simulink model "motor_control_model_mk4"  (R2023b)
settings: Solver=FixedStepAuto  StartTime=0.0  StopTime=80  FixedStep=0.0001  RelTol=1e-5
values from neighbouring files (symbols this model uses):
  A = 1    [paramterters.mat]    (also in set_parameters.m)
  batt_volt = 144    [paramterters.mat]    (also in set_parameters.m)
  C_d = 0.7    [paramterters.mat]    (also in set_parameters.m)
  fric_coeff = 0.03    [paramterters.mat]    (also in set_parameters.m)
  g = 9.81    [paramterters.mat]    (also in set_parameters.m)
  gear_ratio = 4.2    [paramterters.mat]    (also in set_parameters.m)
  grad_degrees = 0    [paramterters.mat]    (also in set_parameters.m)
  J_net = 1.34126984127    [paramterters.mat]    (also in set_parameters.m)
  K_t = 0.3472    [paramterters.mat]    (also in set_parameters.m)
  mass_vehicle = 350    [paramterters.mat]    (also in set_parameters.m)
  motor_eff = 0.85    [paramterters.mat]    (also in set_parameters.m)
  pc_eff = 0.9    [paramterters.mat]    (also in set_parameters.m)
  R_a = 0.02    [paramterters.mat]    (also in set_parameters.m)
  rho = 1.29    [paramterters.mat]    (also in set_parameters.m)
  wheel_radius = 0.26    [paramterters.mat]    (also in set_parameters.m)
libraries: slpidlib x3, spsPWMGeneratorDCDCLib x1
settings Model: Creator=shank  LastModifiedBy=shank

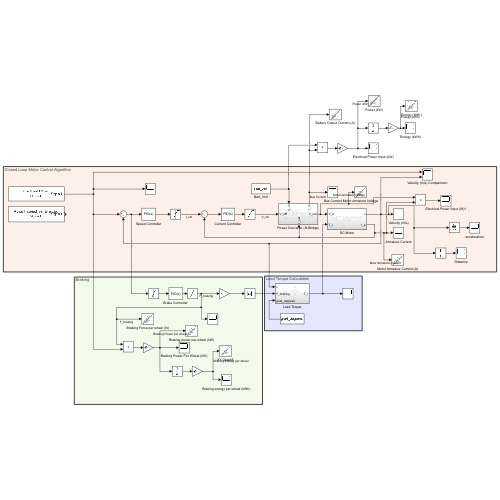
[thumbnail: Simulink's stored preview of the top-level diagram]
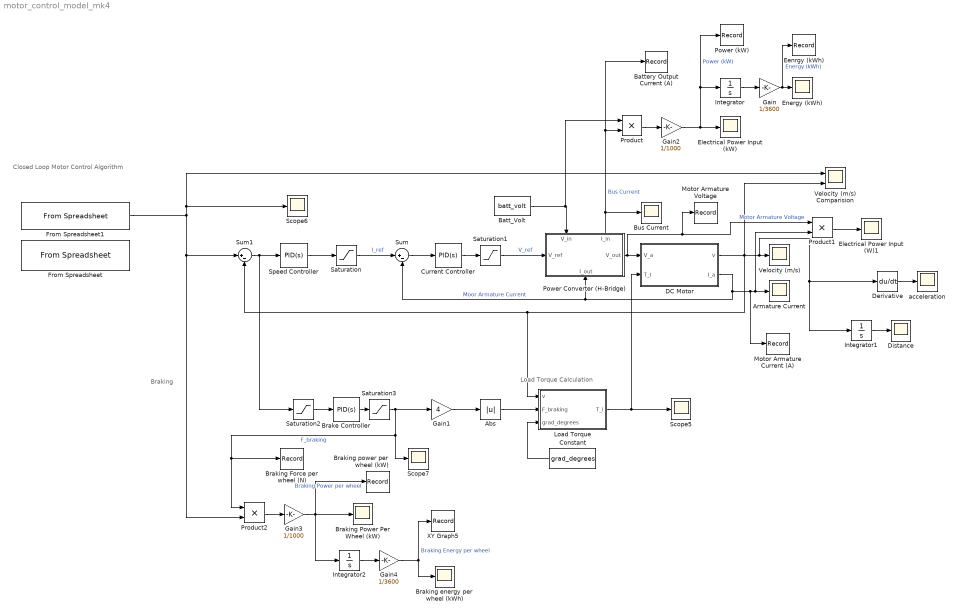
== system motor_control_model_mk4 ==
  note: Closed Loop Motor Control Algorithm
  note: Load Torque Calculation
  note: Braking
  Abs : Abs  SaturateOnIntegerOverflow=off
  Armature Current : Scope
  Batt_Volt : Constant  Value=batt_volt
  Battery Output Current (A) : Record  FileSettingsInternal="{\"entries\":[{\"content\":{\"excelSettings\":{\"content\":{},\"type\":\"Streamout.ExcelSettings\"}},\"type\":\"Streamout.FileSettingStorage\",\"uuid\":\"\"}],\"packageUris\":[\"http:\\/\\/schema.mathworks.com\\/mf0\\/streamout_blocks\\/R2020a\"],\"version\":\"1.0\"}"  Layout=[1 1]  SignalsInternal="{\"entries\":[{\"content\":{\"signals\":[{\"content\":{\"blockPath\":[],\"dimensions\":[1],\"domain\":\"\",\"lineColor\":\"#77ac30\",\"plots\":[1],\"port\":1,\"sid\":[\"\"],\"signalID\":369,\"signalName\":\"Bus Current\"},\"type\":\"RecordBlkView.Signal\",\"uuid\":\"\"}]},\"type\":\"RecordBlkView.InputSignals\",\"uuid\":\"\"}],\"packageUris\":[\"http:\\/\\/schema.mathworks.com\\/mf0\\/streamout_blocks\\/R2020a\"],\"version\":\"1.0\"}"  CompatibilityTag=XY
  Brake Controller : slpidlib/PID Controller  Controller=PID  Form=Parallel  TimeDomain=Continuous-time  UseExternalTs=off  SampleTime=-1  IntegratorMethod=Forward Euler  FilterMethod=Forward Euler  ControllerParametersSource=internal  P=500  I=0  UseKiTs=off  D=10  N=100  UseFilter=on  TunerSelectOption=Transfer Function Based (PID Tuner App)  InitialConditionSource=internal  InitialConditionForIntegrator=0  InitialConditionForFilter=0  DifferentiatorICPrevScaledInput=0  ExternalReset=none  TrackingMode=off  Kt=1  LimitOutput=off  SatLimitsSource=internal  UpperSaturationLimit=inf  LowerSaturationLimit=-inf  LinearizeAsGain=on  AntiWindupMode=none  Kb=1  LimitIntegrator=off  UpperIntegratorSaturationLimit=inf  LowerIntegratorSaturationLimit=-inf  POutMin=[]  POutMax=[]  IOutMin=[]  IOutMax=[]  DOutMin=[]  DOutMax=[]  NOutMin=[]  NOutMax=[]  SumOutMin=[]  SumOutMax=[]  SaturationOutMin=[]  SaturationOutMax=[]  PParamMin=[]  PParamMax=[]  IParamMin=[]  IParamMax=[]  DParamMin=[]  DParamMax=[]  NParamMin=[]  NParamMax=[]  KbParamMin=[]  KbParamMax=[]  KtParamMin=[]  KtParamMax=[]  KbOutMin=[]  KbOutMax=[]  KtOutMin=[]  KtOutMax=[]  IntegratorOutMin=[]  IntegratorOutMax=[]  FilterOutMin=[]  FilterOutMax=[]  SumI1OutMin=[]  SumI1OutMax=[]  SumI2OutMin=[]  SumI2OutMax=[]  SumI3OutMin=[]  SumI3OutMax=[]  SumI4OutMin=[]  SumI4OutMax=[]  SumDOutMin=[]  SumDOutMax=[]  DifferentiatorOutMin=[]  DifferentiatorOutMax=[]  FilterDiffOutCoefMin=[]  FilterDiffOutCoefMax=[]  ReciprocalOutMin=[]  ReciprocalOutMax=[]  SumDenOutMin=[]  SumDenOutMax=[]  SumNumOutMin=[]  SumNumOutMax=[]  DivideOutMin=[]  DivideOutMax=[]  UdiffTsProdOutMin=[]  UdiffTsProdOutMax=[]  NTsProdOutMin=[]  NTsProdOutMax=[]  UintegralTsProdOutMin=[]  UintegralTsProdOutMax=[]  UngainTsProdOutMin=[]  UngainTsProdOutMax=[]  ClampingZeroOutDataTypeStr=Inherit: Inherit via back propagation  ClampingZeroOutMin=[]  ClampingZeroOutMax=[]  FilterDenConstantOutDataTypeStr=Inherit: Inherit via back propagation  FilterDenConstantOutMin=[]  FilterDenConstantOutMax=[]  PCopyOutDataTypeStr=Inherit: Inherit via back propagation  PCopyOutMin=[]  PCopyOutMax=[]  NCopyOutDataTypeStr=Inherit: Inherit via back propagation  NCopyOutMin=[]  NCopyOutMax=[]  IntegratorContinuousStateAttributes=''  IntegratorStateMustResolveToSignalObject=off  IntegratorRTWStateStorageClass=Auto  FilterContinuousStateAttributes=''  FilterStateMustResolveToSignalObject=off  FilterRTWStateStorageClass=Auto  ParallelPVariant=InternalParameters  IdealPVariant=Disabled  IVariant=InternalParameters  DVariant=InternalParameters  IntegratorVariant=Continuous  SatVariant=Disabled  AWVariant=Passthrough  PCopyVariant=Disabled  TRVariant=Disabled  FdbkBlocksVariant=Forward  IdealPFdbkVariant=Disabled  SatFdbkVariant=Disabled  DerivativeFilterVariant=ContFilter  NVariant=InternalParameters  NCopyVariant=Disabled  FilterICVariant=InternalICsFilter  IntegratorICVariant=InternalICs  ExternalResetVariant=Disabled  TRSumVariant=Passthrough  SumFdbkVariant=Disabled  SumVariant=Sum_PID  TsampFilterVariant=InternalTs  TsampNgainVariant=Passthrough  TsampIntegralVariant=Disabled_SignalSpec  ExternalSaturationOutDataTypeStr=Inherit: Same as second input
  Braking Force per wheel (N) : Record  FileSettingsInternal="{\"entries\":[{\"content\":{\"excelSettings\":{\"content\":{},\"type\":\"Streamout.ExcelSettings\"}},\"type\":\"Streamout.FileSettingStorage\",\"uuid\":\"\"}],\"packageUris\":[\"http:\\/\\/schema.mathworks.com\\/mf0\\/streamout_blocks\\/R2020a\"],\"version\":\"1.0\"}"  Layout=[1 1]  SignalsInternal="{\"entries\":[{\"content\":{\"signals\":[{\"content\":{\"blockPath\":[],\"dimensions\":[1],\"domain\":\"\",\"lineColor\":\"#4dbeee\",\"plots\":[1],\"port\":1,\"sid\":[\"\"],\"signalID\":373,\"signalName\":\"F_braking\"},\"type\":\"RecordBlkView.Signal\",\"uuid\":\"\"}]},\"type\":\"RecordBlkView.InputSignals\",\"uuid\":\"\"}],\"packageUris\":[\"http:\\/\\/schema.mathworks.com\\/mf0\\/streamout_blocks\\/R2020a\"],\"version\":\"1.0\"}"  CompatibilityTag=XY
  Braking Power Per Wheel (kW) : Scope
  Braking energy per wheel (kWh) : Scope
  Braking power per wheel (kW) : Record  FileSettingsInternal="{\"entries\":[{\"content\":{\"excelSettings\":{\"content\":{},\"type\":\"Streamout.ExcelSettings\"}},\"type\":\"Streamout.FileSettingStorage\",\"uuid\":\"\"}],\"packageUris\":[\"http:\\/\\/schema.mathworks.com\\/mf0\\/streamout_blocks\\/R2020a\"],\"version\":\"1.0\"}"  Layout=[1 1]  SignalsInternal="{\"entries\":[{\"content\":{\"signals\":[{\"content\":{\"blockPath\":[],\"dimensions\":[1],\"domain\":\"\",\"lineColor\":\"#a2142f\",\"plots\":[1],\"port\":1,\"sid\":[\"\"],\"signalID\":377,\"signalName\":\"Braking Power per wheel\"},\"type\":\"RecordBlkView.Signal\",\"uuid\":\"\"}]},\"type\":\"RecordBlkView.InputSignals\",\"uuid\":\"\"}],\"packageUris\":[\"http:\\/\\/schema.mathworks.com\\/mf0\\/streamout_blocks\\/R2020a\"],\"version\":\"1.0\"}"  CompatibilityTag=XY
  Bus Current : Scope
  Constant : Constant  Value=grad_degrees
  Current Controller : slpidlib/PID Controller  Controller=PID  Form=Parallel  TimeDomain=Continuous-time  UseExternalTs=off  SampleTime=-1  IntegratorMethod=Forward Euler  FilterMethod=Forward Euler  ControllerParametersSource=internal  P=500  I=0  UseKiTs=off  D=10  N=100  UseFilter=on  TunerSelectOption=Transfer Function Based (PID Tuner App)  InitialConditionSource=internal  InitialConditionForIntegrator=0  InitialConditionForFilter=0  DifferentiatorICPrevScaledInput=0  ExternalReset=none  TrackingMode=off  Kt=1  LimitOutput=off  SatLimitsSource=internal  UpperSaturationLimit=inf  LowerSaturationLimit=-inf  LinearizeAsGain=on  AntiWindupMode=none  Kb=1  LimitIntegrator=off  UpperIntegratorSaturationLimit=inf  LowerIntegratorSaturationLimit=-inf  POutMin=[]  POutMax=[]  IOutMin=[]  IOutMax=[]  DOutMin=[]  DOutMax=[]  NOutMin=[]  NOutMax=[]  SumOutMin=[]  SumOutMax=[]  SaturationOutMin=[]  SaturationOutMax=[]  PParamMin=[]  PParamMax=[]  IParamMin=[]  IParamMax=[]  DParamMin=[]  DParamMax=[]  NParamMin=[]  NParamMax=[]  KbParamMin=[]  KbParamMax=[]  KtParamMin=[]  KtParamMax=[]  KbOutMin=[]  KbOutMax=[]  KtOutMin=[]  KtOutMax=[]  IntegratorOutMin=[]  IntegratorOutMax=[]  FilterOutMin=[]  FilterOutMax=[]  SumI1OutMin=[]  SumI1OutMax=[]  SumI2OutMin=[]  SumI2OutMax=[]  SumI3OutMin=[]  SumI3OutMax=[]  SumI4OutMin=[]  SumI4OutMax=[]  SumDOutMin=[]  SumDOutMax=[]  DifferentiatorOutMin=[]  DifferentiatorOutMax=[]  FilterDiffOutCoefMin=[]  FilterDiffOutCoefMax=[]  ReciprocalOutMin=[]  ReciprocalOutMax=[]  SumDenOutMin=[]  SumDenOutMax=[]  SumNumOutMin=[]  SumNumOutMax=[]  DivideOutMin=[]  DivideOutMax=[]  UdiffTsProdOutMin=[]  UdiffTsProdOutMax=[]  NTsProdOutMin=[]  NTsProdOutMax=[]  UintegralTsProdOutMin=[]  UintegralTsProdOutMax=[]  UngainTsProdOutMin=[]  UngainTsProdOutMax=[]  ClampingZeroOutDataTypeStr=Inherit: Inherit via back propagation  ClampingZeroOutMin=[]  ClampingZeroOutMax=[]  FilterDenConstantOutDataTypeStr=Inherit: Inherit via back propagation  FilterDenConstantOutMin=[]  FilterDenConstantOutMax=[]  PCopyOutDataTypeStr=Inherit: Inherit via back propagation  PCopyOutMin=[]  PCopyOutMax=[]  NCopyOutDataTypeStr=Inherit: Inherit via back propagation  NCopyOutMin=[]  NCopyOutMax=[]  IntegratorContinuousStateAttributes=''  IntegratorStateMustResolveToSignalObject=off  IntegratorRTWStateStorageClass=Auto  FilterContinuousStateAttributes=''  FilterStateMustResolveToSignalObject=off  FilterRTWStateStorageClass=Auto  ParallelPVariant=InternalParameters  IdealPVariant=Disabled  IVariant=InternalParameters  DVariant=InternalParameters  IntegratorVariant=Continuous  SatVariant=Disabled  AWVariant=Passthrough  PCopyVariant=Disabled  TRVariant=Disabled  FdbkBlocksVariant=Forward  IdealPFdbkVariant=Disabled  SatFdbkVariant=Disabled  DerivativeFilterVariant=ContFilter  NVariant=InternalParameters  NCopyVariant=Disabled  FilterICVariant=InternalICsFilter  IntegratorICVariant=InternalICs  ExternalResetVariant=Disabled  TRSumVariant=Passthrough  SumFdbkVariant=Disabled  SumVariant=Sum_PID  TsampFilterVariant=InternalTs  TsampNgainVariant=Passthrough  TsampIntegralVariant=Disabled_SignalSpec  ExternalSaturationOutDataTypeStr=Inherit: Same as second input
  DC Motor : Subsystem
  Derivative : Derivative
  Distance : Scope
  Eenrgy (kWh) : Record  FileSettingsInternal="{\"entries\":[{\"content\":{\"excelSettings\":{\"content\":{},\"type\":\"Streamout.ExcelSettings\"}},\"type\":\"Streamout.FileSettingStorage\",\"uuid\":\"\"}],\"packageUris\":[\"http:\\/\\/schema.mathworks.com\\/mf0\\/streamout_blocks\\/R2020a\"],\"version\":\"1.0\"}"  Layout=[1 1]  SignalsInternal="{\"entries\":[{\"content\":{\"signals\":[{\"content\":{\"blockPath\":[],\"dimensions\":[1],\"domain\":\"\",\"lineColor\":\"#139fff\",\"port\":1,\"sid\":[\"\"],\"signalID\":381,\"signalName\":\"Energy (kWh)\"},\"type\":\"RecordBlkView.Signal\",\"uuid\":\"\"}]},\"type\":\"RecordBlkView.InputSignals\",\"uuid\":\"\"}],\"packageUris\":[\"http:\\/\\/schema.mathworks.com\\/mf0\\/streamout_blocks\\/R2020a\"],\"version\":\"1.0\"}"  VisualizationBindings="{\"xyplotplugin\":{\"info\":[{\"series\":[],\"subplotID\":1}]}}"  CompatibilityTag=XY
  Electrical Power Input (W)1 : Scope
  Electrical Power Input (kW) : Scope
  Energy (kWh) : Scope
  From Spreadsheet : FromSpreadsheet  FileName=Adyant_speed_vs_time.xlsx  Range=A1:B4138  ExtrapolationBeforeFirstDataPoint=Ground value  ExtrapolationAfterLastDataPoint=Ground value
  From Spreadsheet1 : FromSpreadsheet  FileName=JonathanLTS.xlsx  Range=A1:B9750  ExtrapolationBeforeFirstDataPoint=Ground value  ExtrapolationAfterLastDataPoint=Ground value
  Gain : Gain  Gain=1/3600
  Gain1 : Gain  Gain=4
  Gain2 : Gain  Gain=1/1000
  Gain3 : Gain  Gain=1/1000
  Gain4 : Gain  Gain=1/3600
  Integrator : Integrator
  Integrator1 : Integrator
  Integrator2 : Integrator
  Load Torque : Subsystem
  Motor Armature Current (A) : Record  FileSettingsInternal="{\"entries\":[{\"content\":{\"excelSettings\":{\"content\":{},\"type\":\"Streamout.ExcelSettings\"}},\"type\":\"Streamout.FileSettingStorage\",\"uuid\":\"\"}],\"packageUris\":[\"http:\\/\\/schema.mathworks.com\\/mf0\\/streamout_blocks\\/R2020a\"],\"version\":\"1.0\"}"  Layout=[1 1]  SignalsInternal="{\"entries\":[{\"content\":{\"signals\":[{\"content\":{\"blockPath\":[],\"dimensions\":[1],\"domain\":\"\",\"lineColor\":\"#ff6929\",\"plots\":[1],\"port\":1,\"sid\":[\"\"],\"signalID\":385,\"signalName\":\"Moor Armature Current\"},\"type\":\"RecordBlkView.Signal\",\"uuid\":\"\"}]},\"type\":\"RecordBlkView.InputSignals\",\"uuid\":\"\"}],\"packageUris\":[\"http:\\/\\/schema.mathworks.com\\/mf0\\/streamout_blocks\\/R2020a\"],\"version\":\"1.0\"}"  CompatibilityTag=XY
  Motor Armature Voltage : Record  FileSettingsInternal="{\"entries\":[{\"content\":{\"excelSettings\":{\"content\":{},\"type\":\"Streamout.ExcelSettings\"}},\"type\":\"Streamout.FileSettingStorage\",\"uuid\":\"\"}],\"packageUris\":[\"http:\\/\\/schema.mathworks.com\\/mf0\\/streamout_blocks\\/R2020a\"],\"version\":\"1.0\"}"  Layout=[1 1]  SignalsInternal="{\"entries\":[{\"content\":{\"signals\":[{\"content\":{\"blockPath\":[],\"dimensions\":[1],\"domain\":\"\",\"lineColor\":\"#b746ff\",\"plots\":[1],\"port\":1,\"sid\":[\"\"],\"signalID\":389,\"signalName\":\"Motor Armature Voltage\"},\"type\":\"RecordBlkView.Signal\",\"uuid\":\"\"}]},\"type\":\"RecordBlkView.InputSignals\",\"uuid\":\"\"}],\"packageUris\":[\"http:\\/\\/schema.mathworks.com\\/mf0\\/streamout_blocks\\/R2020a\"],\"version\":\"1.0\"}"  CompatibilityTag=XY
  Power (kW) : Record  FileSettingsInternal="{\"entries\":[{\"content\":{\"excelSettings\":{\"content\":{},\"type\":\"Streamout.ExcelSettings\"}},\"type\":\"Streamout.FileSettingStorage\",\"uuid\":\"\"}],\"packageUris\":[\"http:\\/\\/schema.mathworks.com\\/mf0\\/streamout_blocks\\/R2020a\"],\"version\":\"1.0\"}"  Layout=[1 1]  SignalsInternal="{\"entries\":[{\"content\":{\"signals\":[{\"content\":{\"blockPath\":[],\"dimensions\":[1],\"domain\":\"\",\"lineColor\":\"#64d413\",\"plots\":[1],\"port\":1,\"sid\":[\"\"],\"signalID\":393,\"signalName\":\"Power (kW)\"},\"type\":\"RecordBlkView.Signal\",\"uuid\":\"\"}]},\"type\":\"RecordBlkView.InputSignals\",\"uuid\":\"\"}],\"packageUris\":[\"http:\\/\\/schema.mathworks.com\\/mf0\\/streamout_blocks\\/R2020a\"],\"version\":\"1.0\"}"  CompatibilityTag=XY
  Power Converter (H-Bridge) : Subsystem
      settings: PortSchema="{\"entries\":[{\"content\":{\"sides\":[{\"content\":{\"connectorIds\":[\"In1\"]},\"type\":\"ConnectorPlacement.EquallySpacedRectSide\",\"uuid\":\"49fd6f3d-18dd-41fa-bf0c-c003bf535265\"},{\"content\":{\"connectorIds\":[\"Out1\"],\"side\":\"RIGHT\"},\"type\":\"ConnectorPlacement.EquallySpacedRectSide\",\"uuid\":\"2112719f-50f6-4c23-b95a-5a4275cbef6d\"},{\"content\":{\"connectorIds\":[\"In2\",\"Out2\"],\"side\":\"TOP\"},\"type\":\"ConnectorPlacement.EquallySpacedRectSide\",\"uuid\":\"ad61c6c3-24f3-4e53-9a57-35f09eeda4ff\"},{\"content\":{\"connectorIds\":[\"In3\"],\"side\":\"BOTTOM\"},\"type\":\"ConnectorPlacement.EquallySpacedRectSide\",\"uuid\":\"a5665d7a-3abb-4f23-830a-cc87f7b6d78e\"}]},\"type\":\"ConnectorPlacement.EquallySpacedConnector\",\"uuid\":\"b12a2cb6-f662-4051-987e-df9392a72524\"}],\"packageUris\":[\"http://schema.mathworks.com/mf0/Connector/R2020b\"],\"version\":\"1.0\"}"
  Product : Product
  Product1 : Product
  Product2 : Product
  Saturation : Saturate  UpperLimit=400  LowerLimit=0
  Saturation1 : Saturate  UpperLimit=144  LowerLimit=0
  Saturation2 : Saturate  UpperLimit=0  LowerLimit=-30
  Saturation3 : Saturate  UpperLimit=0  LowerLimit=-1800
  Scope5 : Scope
  Scope6 : Scope
  Scope7 : Scope
  Speed Controller : slpidlib/PID Controller  Controller=PID  Form=Parallel  TimeDomain=Continuous-time  UseExternalTs=off  SampleTime=-1  IntegratorMethod=Forward Euler  FilterMethod=Forward Euler  ControllerParametersSource=internal  P=300  I=0  UseKiTs=off  D=0  N=100  UseFilter=on  TunerSelectOption=Transfer Function Based (PID Tuner App)  InitialConditionSource=internal  InitialConditionForIntegrator=0  InitialConditionForFilter=0  DifferentiatorICPrevScaledInput=0  ExternalReset=none  TrackingMode=off  Kt=1  LimitOutput=off  SatLimitsSource=internal  UpperSaturationLimit=inf  LowerSaturationLimit=-inf  LinearizeAsGain=on  AntiWindupMode=none  Kb=1  LimitIntegrator=off  UpperIntegratorSaturationLimit=inf  LowerIntegratorSaturationLimit=-inf  POutMin=[]  POutMax=[]  IOutMin=[]  IOutMax=[]  DOutMin=[]  DOutMax=[]  NOutMin=[]  NOutMax=[]  SumOutMin=[]  SumOutMax=[]  SaturationOutMin=[]  SaturationOutMax=[]  PParamMin=[]  PParamMax=[]  IParamMin=[]  IParamMax=[]  DParamMin=[]  DParamMax=[]  NParamMin=[]  NParamMax=[]  KbParamMin=[]  KbParamMax=[]  KtParamMin=[]  KtParamMax=[]  KbOutMin=[]  KbOutMax=[]  KtOutMin=[]  KtOutMax=[]  IntegratorOutMin=[]  IntegratorOutMax=[]  FilterOutMin=[]  FilterOutMax=[]  SumI1OutMin=[]  SumI1OutMax=[]  SumI2OutMin=[]  SumI2OutMax=[]  SumI3OutMin=[]  SumI3OutMax=[]  SumI4OutMin=[]  SumI4OutMax=[]  SumDOutMin=[]  SumDOutMax=[]  DifferentiatorOutMin=[]  DifferentiatorOutMax=[]  FilterDiffOutCoefMin=[]  FilterDiffOutCoefMax=[]  ReciprocalOutMin=[]  ReciprocalOutMax=[]  SumDenOutMin=[]  SumDenOutMax=[]  SumNumOutMin=[]  SumNumOutMax=[]  DivideOutMin=[]  DivideOutMax=[]  UdiffTsProdOutMin=[]  UdiffTsProdOutMax=[]  NTsProdOutMin=[]  NTsProdOutMax=[]  UintegralTsProdOutMin=[]  UintegralTsProdOutMax=[]  UngainTsProdOutMin=[]  UngainTsProdOutMax=[]  ClampingZeroOutDataTypeStr=Inherit: Inherit via back propagation  ClampingZeroOutMin=[]  ClampingZeroOutMax=[]  FilterDenConstantOutDataTypeStr=Inherit: Inherit via back propagation  FilterDenConstantOutMin=[]  FilterDenConstantOutMax=[]  PCopyOutDataTypeStr=Inherit: Inherit via back propagation  PCopyOutMin=[]  PCopyOutMax=[]  NCopyOutDataTypeStr=Inherit: Inherit via back propagation  NCopyOutMin=[]  NCopyOutMax=[]  IntegratorContinuousStateAttributes=''  IntegratorStateMustResolveToSignalObject=off  IntegratorRTWStateStorageClass=Auto  FilterContinuousStateAttributes=''  FilterStateMustResolveToSignalObject=off  FilterRTWStateStorageClass=Auto  ParallelPVariant=InternalParameters  IdealPVariant=Disabled  IVariant=InternalParameters  DVariant=InternalParameters  IntegratorVariant=Continuous  SatVariant=Disabled  AWVariant=Passthrough  PCopyVariant=Disabled  TRVariant=Disabled  FdbkBlocksVariant=Forward  IdealPFdbkVariant=Disabled  SatFdbkVariant=Disabled  DerivativeFilterVariant=ContFilter  NVariant=InternalParameters  NCopyVariant=Disabled  FilterICVariant=InternalICsFilter  IntegratorICVariant=InternalICs  ExternalResetVariant=Disabled  TRSumVariant=Passthrough  SumFdbkVariant=Disabled  SumVariant=Sum_PID  TsampFilterVariant=InternalTs  TsampNgainVariant=Passthrough  TsampIntegralVariant=Disabled_SignalSpec  ExternalSaturationOutDataTypeStr=Inherit: Same as second input
  Sum : Sum  Inputs=|+-
  Sum1 : Sum  Inputs=|+-
  Velocity (m/s) : Scope
  Velocity (m/s) Comparision : Scope  NumInputPorts=2
  XY Graph5 : Record  FileSettingsInternal="{\"entries\":[{\"content\":{\"excelSettings\":{\"content\":{},\"type\":\"Streamout.ExcelSettings\"}},\"type\":\"Streamout.FileSettingStorage\",\"uuid\":\"\"}],\"packageUris\":[\"http:\\/\\/schema.mathworks.com\\/mf0\\/streamout_blocks\\/R2020a\"],\"version\":\"1.0\"}"  Layout=[1 1]  SignalsInternal="{\"entries\":[{\"content\":{\"signals\":[{\"content\":{\"blockPath\":[],\"dimensions\":[1],\"domain\":\"\",\"lineColor\":\"#a2142f\",\"plots\":[1],\"port\":1,\"sid\":[\"\"],\"signalID\":397,\"signalName\":\"Braking Energy per wheel\"},\"type\":\"RecordBlkView.Signal\",\"uuid\":\"\"}]},\"type\":\"RecordBlkView.InputSignals\",\"uuid\":\"\"}],\"packageUris\":[\"http:\\/\\/schema.mathworks.com\\/mf0\\/streamout_blocks\\/R2020a\"],\"version\":\"1.0\"}"  VisualizationBindings="{\"xyplotplugin\":{\"info\":[{\"series\":[{\"bindingParametersList\":[{\"parameter\":\"X-Axis\",\"signalID\":397,\"signalName\":\"Braking Energy per wheel\"}],\"seriesID\":43690}],\"subplotID\":1}]}}"  CompatibilityTag=XY
  acceleration : Scope
  wires:
  Speed Controller/1 -> Saturation/1
  Current Controller/1 -> Saturation1/1
  Saturation/1 -> Sum/1  "I_ref"
  Sum/1 -> Current Controller/1
  Sum1/1 -> Saturation2/1, Speed Controller/1
  From Spreadsheet1/1 -> Sum1/1, Product2/2, Velocity (m/s) Comparision/1, Scope6/1
  Power Converter (H-Bridge)/1(V_out) -> DC Motor/1(V_a), Product1/1, Motor Armature Voltage/1  "Motor Armature Voltage"
  Saturation1/1 -> Power Converter (H-Bridge)/1(V_ref)  "V_ref"
  DC Motor/2(I_a) -> Product1/2, Armature Current/1, Motor Armature Current (A)/1, Sum/2, Power Converter (H-Bridge)/3(I_out)  "Moor Armature Current"
  DC Motor/1(v) -> Sum1/2, Load Torque/1(v), Velocity (m/s) Comparision/2, Integrator1/1, Derivative/1, Velocity (m/s)/1
  Power Converter (H-Bridge)/2(I_in) -> Product/2, Battery Output Current (A)/1, Bus Current/1  "Bus Current"
  Batt_Volt/1 -> Product/1, Power Converter (H-Bridge)/2(V_in)
  Product/1 -> Gain2/1
  Constant/1 -> Load Torque/3(grad_degrees)
  Load Torque/1(T_l) -> DC Motor/2(T_l), Scope5/1
  Saturation2/1 -> Brake Controller/1
  Brake Controller/1 -> Saturation3/1
  Saturation3/1 -> Scope7/1, Product2/1, Braking Force per wheel (N)/1, Gain1/1  "F_braking"
  Integrator/1 -> Gain/1
  Gain/1 -> Eenrgy (kWh)/1, Energy (kWh)/1  "Energy (kWh)"
  Product1/1 -> Electrical Power Input (W)1/1
  Derivative/1 -> acceleration/1
  Integrator1/1 -> Distance/1
  Abs/1 -> Load Torque/2(F_braking)
  Gain1/1 -> Abs/1
  Gain2/1 -> Power (kW)/1, Integrator/1, Electrical Power Input (kW)/1  "Power (kW)"
  Product2/1 -> Gain3/1
  Gain3/1 -> Braking power per wheel (kW)/1, Integrator2/1, Braking Power Per Wheel (kW)/1  "Braking Power per wheel"
  Gain4/1 -> Braking energy per wheel (kWh)/1, XY Graph5/1  "Braking Energy per wheel"
  Integrator2/1 -> Gain4/1

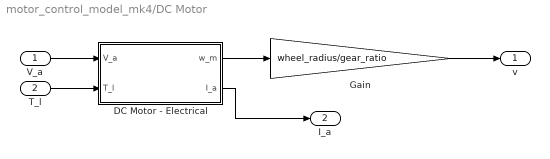
== system motor_control_model_mk4/DC Motor ==
  V_a : Inport
  T_l : Inport  Port=2
  DC Motor - Electrical : Subsystem
  Gain : Gain  Gain=wheel_radius/gear_ratio
  v : Outport
  I_a : Outport  Port=2
  wires:
  DC Motor - Electrical/1(w_m) -> Gain/1
  V_a/1 -> DC Motor - Electrical/1(V_a)
  Gain/1 -> v/1
  DC Motor - Electrical/2(I_a) -> I_a/1
  T_l/1 -> DC Motor - Electrical/2(T_l)

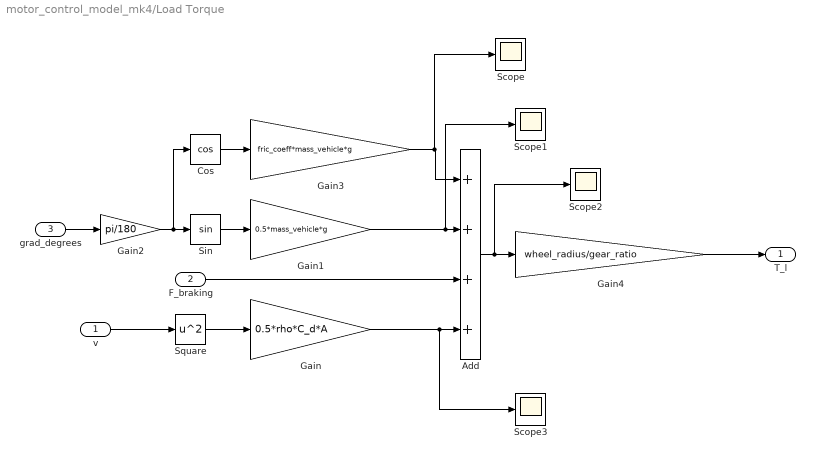
== system motor_control_model_mk4/Load Torque ==
  v : Inport
  F_braking : Inport  Port=2
  grad_degrees : Inport  Port=3
  Add : Sum  Inputs=++++
  Cos : Trigonometry  Operator=cos
  Gain : Gain  Gain=0.5*rho*C_d*A
  Gain1 : Gain  Gain=0.5*mass_vehicle*g
  Gain2 : Gain  Gain=pi/180
  Gain3 : Gain  Gain=fric_coeff*mass_vehicle*g
  Gain4 : Gain  Gain=wheel_radius/gear_ratio
  Scope{,1..3} (4 alike) : Scope
  Sin : Trigonometry
  Square : Math  Operator=square
  T_l : Outport
  wires:
  grad_degrees/1 -> Gain2/1
  Add/1 -> Scope2/1, Gain4/1
  Gain/1 -> Scope3/1, Add/4
  Sin/1 -> Gain1/1
  Gain1/1 -> Scope1/1, Add/2
  Gain4/1 -> T_l/1
  v/1 -> Square/1
  Square/1 -> Gain/1
  Cos/1 -> Gain3/1
  Gain2/1 -> Cos/1, Sin/1
  Gain3/1 -> Scope/1, Add/1
  F_braking/1 -> Add/3

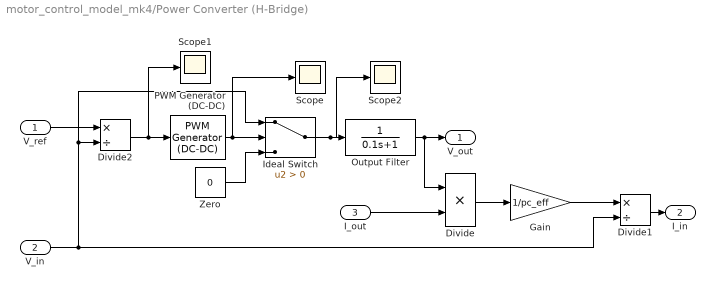
== system motor_control_model_mk4/Power Converter (H-Bridge) ==
  V_ref : Inport
  V_in : Inport  Port=2
  I_out : Inport  Port=3
  Divide : Product  Inputs=**
  Divide1 : Product  Inputs=*/
  Divide2 : Product  Inputs=*/
  Gain : Gain  Gain=1/pc_eff
  Ideal Switch : Switch  Criteria=u2 > Threshold  SaturateOnIntegerOverflow=off  InputSameDT=off
  Output Filter : TransferFcn  Denominator=[0.1 1]
  PWM Generator (DC-DC) : spsPWMGeneratorDCDCLib/PWM Generator (DC-DC)  Fsw=1/25e3  Ts=0
  Scope : Scope
  Scope1 : Scope
  Scope2 : Scope
  Zero : Constant  Value=0  OutDataTypeStr=Inherit: Inherit via back propagation
  V_out : Outport
  I_in : Outport  Port=2
  wires:
  I_out/1 -> Divide/2
  V_in/1 -> Ideal Switch/1, Divide2/2, Divide1/2
  Divide1/1 -> I_in/1
  Divide/1 -> Gain/1
  Gain/1 -> Divide1/1
  V_ref/1 -> Divide2/1
  Divide2/1 -> Scope1/1, PWM Generator (DC-DC)/1
  PWM Generator (DC-DC)/1 -> Scope/1, Ideal Switch/2
  Zero/1 -> Ideal Switch/3
  Output Filter/1 -> Divide/1, V_out/1
  Ideal Switch/1 -> Scope2/1, Output Filter/1

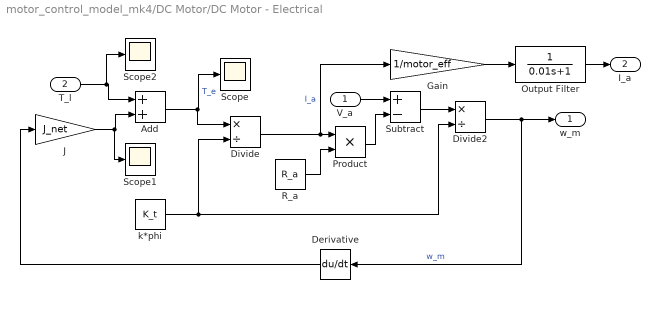
== system motor_control_model_mk4/DC Motor/DC Motor - Electrical ==
  V_a : Inport
  T_l : Inport  Port=2
  Add : Sum
  Derivative : Derivative
  Divide : Product  Inputs=*/
  Divide2 : Product  Inputs=*/
  Gain : Gain  Gain=1/motor_eff
  J : Gain  Gain=J_net
  Output Filter : TransferFcn  Denominator=[0.01 1]
  Product : Product
  R_a : Constant  Value=R_a
  Scope : Scope
  Scope1 : Scope
  Scope2 : Scope
  Subtract : Sum  Inputs=+-
  k*phi : Constant  Value=K_t
  w_m : Outport
  I_a : Outport  Port=2
  wires:
  Divide2/1 -> Derivative/1, w_m/1  "w_m"
  J/1 -> Scope1/1, Add/2
  Divide/1 -> Gain/1, Product/1  "I_a"
  k*phi/1 -> Divide/2, Divide2/2
  Add/1 -> Scope/1, Divide/1  "T_e"
  T_l/1 -> Scope2/1, Add/1
  Subtract/1 -> Divide2/1
  R_a/1 -> Product/2
  Product/1 -> Subtract/2
  V_a/1 -> Subtract/1
  Derivative/1 -> J/1
  Gain/1 -> Output Filter/1
  Output Filter/1 -> I_a/1
